simulink model "Trigggred_Sub_Sys"  (R2016a)
settings: Solver=VariableStepAuto  StartTime=0.0  StopTime=inf  RelTol=1e-3
model workspace (MAT data in the model file):
  cs : Simulink.ConfigSet (value not decoded)
settings Model: Creator=LEGION  LastModifiedBy=LEGION

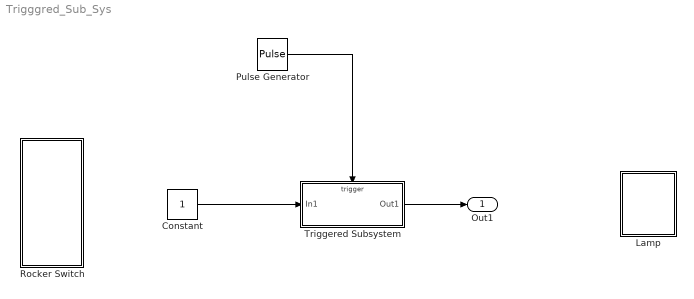
== system Trigggred_Sub_Sys ==
  Constant : Constant
  Lamp : Subsystem  DialogController=hmiCreateDDGDialog  IsWebBlock=on  mask(MWDashboardBlock){webBlockId=65e3e26a-4887-494a-ae41-3a1650a1eaf4, webBlockType=lamp, ShowInLibBrowser=on, ShowInitialText=on, HMISrcModelName=Trigggred_Sub_Sys}
      mask prompts: webBlockType "WebBlock Type"; HMISrcModelName "Source Model"
      mask Help: helpview([docroot '/mapfiles/simulink.map'], 'hmi_lamp')
      mask Display:
      | if strcmp(get_param(bdroot(gcb),'BlockDiagramType'), 'library')
      |     image([(matlabroot) '/toolbox/simulink/hmi/icons/Lamp.png']);
      | end
  Pulse Generator : DiscretePulseGenerator  PulseType=Time based  Period=0.05  PulseWidth=50
  Rocker Switch : Subsystem  DialogController=hmiCreateDDGDialog  IsWebBlock=on  mask(MWDashboardBlock){webBlockId=85520d0e-cdb5-414e-b5da-062de04aeb45, webBlockType=rockerswitch, ShowInLibBrowser=on, ShowInitialText=on, HMISrcModelName=Trigggred_Sub_Sys}
      mask prompts: webBlockId "WebBlock Id"; webBlockType "WebBlock Type"; HMISrcModelName "Source Model"
      mask Help: helpview([docroot '/mapfiles/simulink.map'], 'hmi_rocker_switch')
      mask Display:
      | if strcmp(get_param(bdroot(gcb),'BlockDiagramType'), 'library')
      |     image([(matlabroot) '/toolbox/simulink/hmi/icons/RockerSwitch.png']);
      | end
  Triggered Subsystem : Subsystem  TreatAsAtomicUnit=on
  Out1 : Outport
  wires:
  Triggered Subsystem/1(Out1) -> Out1/1
  Constant/1 -> Triggered Subsystem/1(In1)
  Pulse Generator/1 -> Triggered Subsystem/Trigger

== system Trigggred_Sub_Sys/Lamp ==

== system Trigggred_Sub_Sys/Rocker Switch ==

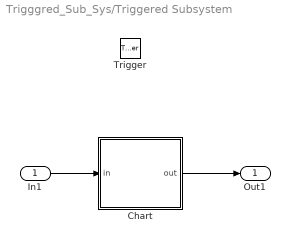
== system Trigggred_Sub_Sys/Triggered Subsystem ==
  In1 : Inport
  Trigger : TriggerPort  TriggerType=either  VariantControl=Variant
  Chart : Stateflow chart  TreatAsAtomicUnit=on
  Out1 : Outport
  wires:
  In1/1 -> Chart/1(in)
  Chart/1(out) -> Out1/1

== stateflow chart Trigggred_Sub_Sys/Triggered Subsystem/Chart ==
  (default) -> (junction 9) : % TurnsOnLamp
  (junction 9) -> (junction 10) [order 1] : [in==1]
  (junction 9) -> (junction 11) [order 2] : {out=0;}
  (junction 10) -> (junction 12) : {out=1;}
  (junction 12) -> (junction 11)
  (junction 11) -> (junction 13)
  data: out output; in input
